simulink model "eml_eqdemo"  (Simulink 6.0)
settings: Solver=FixedStepDiscrete  StartTime=0.0  StopTime=inf  RelTol=1e-3
InitFcn:
  | initsim
undefined symbols (not defined in the file or in its folder): params, qammod
libraries: commsink2 x4, dspsigattribs x4, commchan2 x2, commdigbbndam2 x2, dsparch4 x1, commrandsrc2 x1, dspsnks4 x1, simulink x1
CloseFcn:
  | rtwprivate ssgencode ModelCloseRequest eqdemo
settings Model: RecordCoverage=on  CovMetricSettings=dmw  Creator=The MathWorks Inc.  LastModifiedBy=batserve  ExtModeAutoUpdateStatusClock=off
settings DataIOCC: SignalLoggingName=logsOut
settings OptimizationCC: InlineInvariantSignals=off  LifeSpan=1
settings DebuggingCC: CheckExecutionContextPreStartOutputMsg=on  CheckExecutionContextRuntimeOutputMsg=on  SolverPrmCheckMsg=none
settings HardwareCC: TargetUnknown=on
settings RTWCC: SystemTargetFile=ert.tlc  TemplateMakefile=ert_default_tmf  GenerateReport=on  ProcessScript=ert_make_rtw_hook  LaunchReport=on
settings CodeAppCC: IgnoreCustomStorageClasses=off  MangleLength=5
settings ERTTargetCC: TargetFcnLib=ansi_tfl_tmw.mat  GenFloatMathFcnCalls=ANSI_C  GenerateSampleERTMain=on  SupportContinuousTime=on  SupportNonInlinedSFcns=on  RootIOFormat=Individual Arguments  ERTCustomFileTemplate=example_file_process.tlc  InitialValueSource=Model

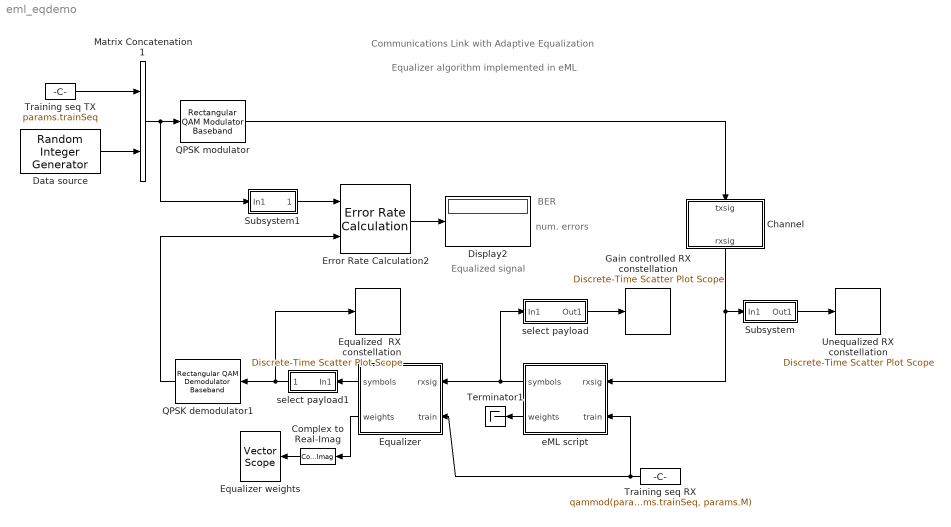
== system eml_eqdemo ==
  note: Communications Link with Adaptive Equalization
  note: Equalizer algorithm implemented in eML
  note: BER
  note: Equalized signal
  note: num. errors
  " Gain controlled RX constellation" : commsink2/Discrete-Time Scatter Plot Scope  Tag=ScatterPlot  sampPerSymb=1  offsetEye=0  numTraces=200  numNewFrames=100  LineMarkers=.  LineColors=b  fading=on  render=on  AxisGrid=on  xMin=-1.84900078842742  xMax=1.93655728027381  yMin=-1.87362349123512  yMax=1.91193457746611  inphaseLabel=In-phase Amplitude  quadratureLabel=Quadrature Amplitude  openScopeAtSimStart=on  FrameNumber=off  FigPos=[261 32 242 242]  figTitle=Scatter Plot  numLinesMax=8  block_type_=scatter
  Channel : Subsystem  Orientation=down  PropExecContextAcrossSSBoundary=on  mask(4-path Rician fading chanel){gain_fade=0+[0 -9 -60 -90], gain_spec=[-10 -60 -60 -60], doppler=0.0001/params.symbolPeriod, SNRdB=60, T=params.symbolPeriod}
      mask prompts: gain_fade "Fading component gains (dB):"; gain_spec "Spectral component gains (dB):"; doppler "Maximum Doppler shift (Hz):"; SNRdB "SNR (dB):"; T "Symbol period (s):"
      mask Display: disp('Rician Fading\nChannel')
  Complex to Real-Imag : ComplexToRealImag  Orientation=left  Output=Real
  Data source : commrandsrc2/Random Integer Generator  mul=4  seed=37  Ts=params.sourcePeriod  frameBased=on  sampPerFrame=params.Nsource  orient=off
  Display2 : Display
  Equalized  RX constellation : commsink2/Discrete-Time Scatter Plot Scope  Tag=ScatterPlot  sampPerSymb=1  offsetEye=0  numTraces=200  numNewFrames=100  LineMarkers=.  LineColors=b  fading=on  render=on  AxisGrid=on  xMin=-1.84900078842742  xMax=1.93655728027381  yMin=-1.87362349123512  yMax=1.91193457746611  inphaseLabel=In-phase Amplitude  quadratureLabel=Quadrature Amplitude  openScopeAtSimStart=on  FrameNumber=off  FigPos=[510 32 242 242]  figTitle=Scatter Plot  numLinesMax=8  block_type_=scatter
  Equalizer : Subsystem  Orientation=left  PropExecContextAcrossSSBoundary=on  mask(Receiver processing (adaptive equalizer)){eqMode=RLS, refTap=4, resetWeights=off}
      mask prompts: eqMode "Adaptive algorithm:"; refTap "Reference tap:"; resetWeights "Reset weights each frame"
      mask init:
      | M = 6; % number of weights
      | mu = 0.025; % step size
      | lambda = 0.99; % forget factor
      | delta1 = 0.1 + 0i; % diagonal element of inv. corr. mtx.
      mask StyleString: popup(LMS|RLS),popup(1|2|3|4|5|6),checkbox
  Equalizer weights : dspsnks4/Vector Scope  Orientation=left  ScopeProperties=off  Domain=User-defined  HorizSpan=1  DisplayProperties=off  AxisGrid=on  Memory=off  FrameNumber=off  AxisLegend=off  AxisZoom=off  OpenScopeAtSimStart=on  OpenScopeImmediately=off  FigPos=[762 31 251 243]  AxisProperties=off  XUnits=Hertz  XRange=[0...Fs/2]  InheritXIncr=off  XIncr=1  XLabel=delay  YUnits=dB  YLabel=Amplitude  LineProperties=off  LineMarkers=.  LineColors=[0 0 1]
      settings: YMin=-2  YMax=2
  Error Rate Calculation2 : commsink2/Error Rate Calculation  N=0  st_delay=0  cp_mode=Entire frame  subframe=[]  PMode=Port  WsName=ErrorVec  RsMode2=off  stop=off  numErr=100  maxBits=1e6
  Matrix Concatenation1 : simulink/Math Operations/Matrix Concatenation  numInports=2  catMethod=Vertical
  QPSK demodulator1 : commdigbbndam2/Rectangular QAM Demodulator Baseband  Orientation=left  M=params.M  OutType=Integer  Dec=Binary  PowType=Min. distance between symbols  MinDist=2  AvgPow=1  PeakPow=1  Ph=0  numSamp=1
  QPSK modulator : commdigbbndam2/Rectangular QAM Modulator Baseband  M=params.M  InType=Integer  Enc=Binary  PowType=Min. distance between symbols  MinDist=2  AvgPow=1  PeakPow=1  Ph=0  numSamp=1
  Subsystem : Subsystem  PropExecContextAcrossSSBoundary=on
      mask Display: disp('Payload')
  Subsystem1 : Subsystem  PropExecContextAcrossSSBoundary=on
      mask Display: disp('Payload')
  Terminator1 : Terminator
  Training seq RX : Constant  Orientation=left  Value=qammod(params.trainSeq, params.M)
  Training seq TX : Constant  Value=params.trainSeq
  Unequalized RX constellation : commsink2/Discrete-Time Scatter Plot Scope  Tag=ScatterPlot  sampPerSymb=1  offsetEye=0  numTraces=500  numNewFrames=50  LineMarkers=.  LineColors=b  fading=on  render=on  AxisGrid=on  xMin=-2  xMax=2  yMin=-2  yMax=2  inphaseLabel=In-phase Amplitude  quadratureLabel=Quadrature Amplitude  openScopeAtSimStart=on  FrameNumber=off  FigPos=[9 32 242 242]  figTitle=Scatter Plot  numLinesMax=8  block_type_=scatter
  eML script : Stateflow chart  Orientation=left  PropExecContextAcrossSSBoundary=on
  select payload : Subsystem  PropExecContextAcrossSSBoundary=on
      mask Display: disp('Payload')
  select payload1 : Subsystem  Orientation=left  PropExecContextAcrossSSBoundary=on
      mask Display: disp('Payload')
  wires:
  Subsystem/1(Out1) -> Unequalized RX constellation/1
  eML script/2(weights) -> Terminator1/1
  Training seq TX/1 -> Matrix Concatenation1/1
  Data source/1 -> Matrix Concatenation1/2
  Matrix Concatenation1/1 -> QPSK modulator/1, Subsystem1/1(In1)
  QPSK modulator/1 -> Channel/1(txsig)
  Subsystem1/1(Out1) -> Error Rate Calculation2/1
  Error Rate Calculation2/1 -> Display2/1
  eML script/1(symbols) -> select payload/1(In1), Equalizer/1(rxsig)
  select payload/1(Out1) -> " Gain controlled RX constellation"/1
  Channel/1(rxsig) -> eML script/1(rxsig), Subsystem/1(In1)
  Training seq RX/1 -> eML script/2(train), Equalizer/2(train)
  Equalizer/1(symbols) -> select payload1/1(In1)
  select payload1/1(Out1) -> QPSK demodulator1/1, Equalized  RX constellation/1
  QPSK demodulator1/1 -> Error Rate Calculation2/2
  Equalizer/2(weights) -> Complex to Real-Imag/1
  Complex to Real-Imag/1 -> Equalizer weights/1

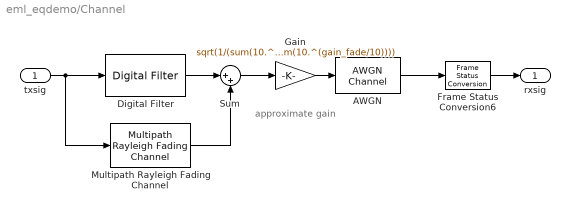
== system eml_eqdemo/Channel ==
  note: approximate gain
  txsig : Inport  Port=1  LatchInput=off
  AWGN : commchan2/AWGN Channel  seed=67  noiseMode="Signal to noise ratio  (SNR)"  EbNodB=10  EsNodB=10  SNRdB=SNRdB  bitsPerSym=1  Ps=1  Tsym=1  variance=1
  Digital Filter : dsparch4/Digital Filter  TypePopup=FIR (all zeros)  IIRFiltStruct=Direct form II transposed  AllPoleFiltStruct=Direct form  FIRFiltStruct=Direct form  CoeffSource=Specify via dialog  NumCoeffs=10.^(gain_spec/20)  DenCoeffs=[1 0.1]  BiQuadCoeffs=[1 0.3 0.4 1 0.1 0.2]  LatticeCoeffs=[0.2 0.4]  denIgnore=on  FiltPerSampPopup=One filter per frame  IC=0  ICnum=0  ICden=0  roundingMode=Floor  overflowMode=off
  Frame Status Conversion6 : dspsigattribs/Frame Status Conversion  growRefPort=off  outframe=Sample-based
  Gain : Gain  Gain=sqrt(1/(sum(10.^(gain_spec/10))+sum(10.^(gain_fade/10))))  SaturateOnIntegerOverflow=on
  Multipath Rayleigh Fading Channel : commchan2/Multipath Rayleigh Fading Channel  Fd=doppler  simTs=T  delayVec=(0:3)*T  gainVecdB=gain_fade  normGain=off  Seed=73
  Sum : Sum  Inputs=|++  SaturateOnIntegerOverflow=on
  rxsig : Outport
  wires:
  AWGN/1 -> Frame Status Conversion6/1
  txsig/1 -> Digital Filter/1, Multipath Rayleigh Fading Channel/1
  Sum/1 -> Gain/1
  Gain/1 -> AWGN/1
  Digital Filter/1 -> Sum/1
  Multipath Rayleigh Fading Channel/1 -> Sum/2
  Frame Status Conversion6/1 -> rxsig/1

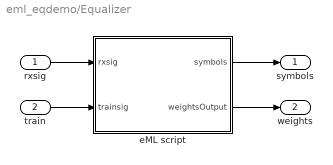
== system eml_eqdemo/Equalizer ==
  rxsig : Inport  Port=1  LatchInput=off
  train : Inport  Port=2  LatchInput=off
  eML script : Stateflow chart  PropExecContextAcrossSSBoundary=on
  symbols : Outport
  weights : Outport  Port=2
  wires:
  eML script/1(symbols) -> symbols/1
  eML script/2(weightsOutput) -> weights/1
  train/1 -> eML script/2(trainsig)
  rxsig/1 -> eML script/1(rxsig)

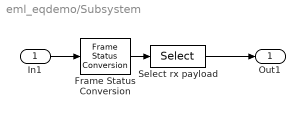
== system eml_eqdemo/Subsystem ==
  In1 : Inport  Port=1  LatchInput=off
  Frame Status Conversion : dspsigattribs/Frame Status Conversion  growRefPort=off  outframe=Frame-based
  Select rx payload : Selector  Elements=(params.Ntrain+1):(params.Nsymbols-10)  InputPortWidth=params.Nsymbols
  Out1 : Outport
  wires:
  In1/1 -> Frame Status Conversion/1
  Select rx payload/1 -> Out1/1
  Frame Status Conversion/1 -> Select rx payload/1

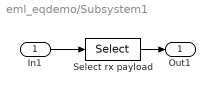
== system eml_eqdemo/Subsystem1 ==
  In1 : Inport  Port=1  LatchInput=off
  Select rx payload : Selector  Elements=(params.Ntrain+1):(params.Nsymbols-10)  InputPortWidth=params.Nsymbols
  Out1 : Outport
  wires:
  In1/1 -> Select rx payload/1
  Select rx payload/1 -> Out1/1

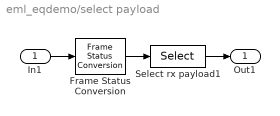
== system eml_eqdemo/select payload ==
  In1 : Inport  Port=1  LatchInput=off
  Frame Status Conversion : dspsigattribs/Frame Status Conversion  growRefPort=off  outframe=Frame-based
  Select rx payload1 : Selector  Elements=(params.Ntrain+1):(params.Nsymbols-10)  InputPortWidth=params.Nsymbols
  Out1 : Outport
  wires:
  Select rx payload1/1 -> Out1/1
  In1/1 -> Frame Status Conversion/1
  Frame Status Conversion/1 -> Select rx payload1/1

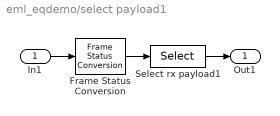
== system eml_eqdemo/select payload1 ==
  In1 : Inport  Port=1  LatchInput=off
  Frame Status Conversion : dspsigattribs/Frame Status Conversion  growRefPort=off  outframe=Frame-based
  Select rx payload1 : Selector  Elements=(params.Ntrain+1):(params.Nsymbols-10)  InputPortWidth=params.Nsymbols
  Out1 : Outport
  wires:
  Frame Status Conversion/1 -> Select rx payload1/1
  In1/1 -> Frame Status Conversion/1
  Select rx payload1/1 -> Out1/1

== matlab function eML script ==
  data: rxsig input double size=250; train input double size=50; symbols output double size=250; weights output double
function [symbols, weights] = gaincontrol(rxsig, train)
% 1-tap adaptive equalizer using LMS or RLS algorithm

% Equalizer settings
lambda = 0.99; % forgetting factor for RLS

% Initialize
Delta = 0.1+0i; % inv. corr. parameter
weights = 0+0i;    

symbols = zeros(length(rxsig),1);
for n = 1:length(rxsig)
    u = rxsig(n);  % received sample
    y = conj(weights) * u;  % output
    if n<=length(train)
        % training mode
        d = train(n);
    else
        % decision-directed mode
        d = detect(real(y)) + 1j*detect(imag(y));
    end
    % Single-tap RLS
    Delta = 1/(lambda/Delta + u*conj(u));
    G = Delta * u;
    e = d - y;  % symbol estimation error
    weights = weights + G*conj(e);  % update weights
    symbols(n) = y;
end


function y = detect(x);
if real(x)<0, y=-1; else y=1; end

== matlab function Equalizer/eML script ==
  data: rxsig input double size=250; trainsig input double size=50; symbols output double size=250; weightsOutput output double size=6; resetWeights parameter double; eqMode parameter double; refTap parameter double; mu parameter double; lambda parameter double; delta1 parameter double
function [symbols, weightsOutput] = equalizer(rxsig, trainsig, resetWeights, eqMode, refTap, mu, lambda, delta1)
% Adaptive equalizer using LMS or RLS algorithm
% By Martin Clark

% Equalizer settings
M = 6; % number of tap weights

persistent weights
if(isempty(weights))
    weights = zeros(M, 1) + 0i;
end

% Initialize
G = zeros(M, 1) + 0i; % Gain vector (both LMS and RLS)
Delta = zeros(M, M) + 0i;  Delta(1:M+1:end) = delta1;  % inv. corr. mtx.
if resetWeights==1
    weights = zeros(M, 1) + 0i;   
end
u = zeros(M, 1) + 0i; % input vector (to tap weights)
delay = refTap - 1;
symbols = zeros(length(rxsig),1);
for n = 1:length(rxsig)
    u = [rxsig(n); u(1:M-1)];  % tapped delay line
    if n >= delay
        y = weights' * u;
        m = n - delay + 1;
        if n<=length(trainsig)
            % training mode
            d = trainsig(m);  
        else
            % decision-directed mode
            d = detect(real(y)) + 1j*detect(imag(y));
        end
        e = d - y;  % symbol estimation error
        if eqMode==1
            % LMS
            G = mu*u;
        else
            % RLS
            G = Delta * u / (lambda + u'*Delta*u);
            Delta = 1/lambda * (Delta - G*u'*Delta);
        end
        weights = weights + G*conj(e);  % update weights
        symbols(m) = y;	% note: last few symbols not estimated
    end
end
weightsOutput = weights;

function y = detect(x)
if real(x)<0, y=-1; else y=1; end
